simulink model "hiptourque"  (R2014b)
settings: Solver=ode3  StartTime=0.0  StopTime=4  FixedStep=.01  RelTol=1e-3
values from neighbouring files (symbols this model uses):
  k = 10    [hip.m]
  p = -phi(end)    [hip.m]
  p1 = (1-cos(phi(end)))*cos(phi(end))*thetadot(end)    [hip.m]
  t1 = cos(phi(end))*thetadot(end)    [hip.m]
settings Model: Creator=hamidreza  LastModifiedBy=hamidreza

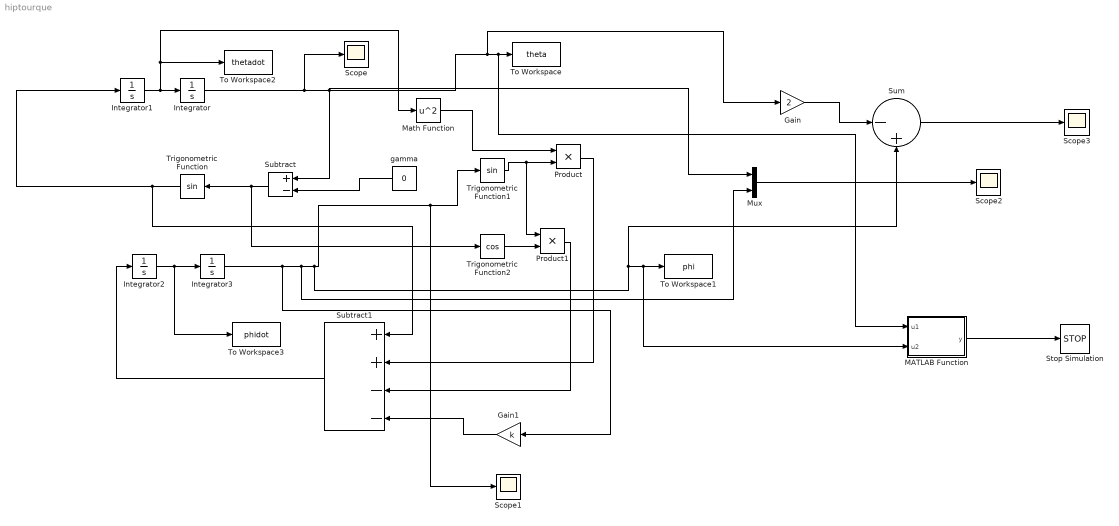
== system hiptourque ==
  Gain : Gain  Gain=2
  Gain1 : Gain  Gain=k
  Integrator : Integrator  InitialCondition=t
  Integrator1 : Integrator  InitialCondition=t1
  Integrator2 : Integrator  InitialCondition=p1
  Integrator3 : Integrator  InitialCondition=p
  MATLAB Function : MATLAB Function  TreatAsAtomicUnit=on
  Math Function : Math  Operator=square  SaturateOnIntegerOverflow=on
  Mux : Mux  Inputs=2
  Product : Product
  Product1 : Product
  Scope{,1..3} (4 alike) : Scope
      Scope1 settings: TimeRange=10  YMin=-1  YMax=1.5
      Scope2 settings: TimeRange=0.66  YMin=-0.2  YMax=0.2  SaveName=ScopeData2
      Scope3 settings: SaveName=ScopeData3
  Stop Simulation : Stop
  Subtract : Sum  Inputs=+-
  Subtract1 : Sum  Inputs=++--
  Sum : Sum  Inputs=|-+
  To Workspace : ToWorkspace  VariableName=theta  SaveFormat=Structure With Time  SampleTime=-1
  To Workspace1 : ToWorkspace  VariableName=phi  SaveFormat=Structure With Time  SampleTime=-1
  To Workspace2 : ToWorkspace  VariableName=thetadot  SaveFormat=Structure With Time  SampleTime=-1
  To Workspace3 : ToWorkspace  VariableName=phidot  SaveFormat=Structure With Time  SampleTime=-1
  Trigonometric Function : Trigonometry  OutputSignalType=real
  Trigonometric Function1 : Trigonometry
  Trigonometric Function2 : Trigonometry  Operator=cos
  "gamma " : Constant  Value=0
  wires:
  Integrator/1 -> Scope/1, Subtract/1, Mux/1, Gain/1, MATLAB Function/1(u1), To Workspace/1
  Trigonometric Function/1 -> Subtract1/1, Integrator1/1
  Integrator1/1 -> Math Function/1, To Workspace2/1, Integrator/1
  Integrator2/1 -> To Workspace3/1, Integrator3/1
  "gamma "/1 -> Subtract/2
  Subtract/1 -> Trigonometric Function2/1, Trigonometric Function/1
  Math Function/1 -> Product/1
  Integrator3/1 -> Gain1/1, Mux/2, Sum/2, MATLAB Function/2(u2), To Workspace1/1, Scope1/1, Trigonometric Function1/1
  Trigonometric Function1/1 -> Product1/1, Product/2
  Product/1 -> Subtract1/2
  Subtract1/1 -> Integrator2/1
  Trigonometric Function2/1 -> Product1/2
  Product1/1 -> Subtract1/3
  Mux/1 -> Scope2/1
  Gain/1 -> Sum/1
  Sum/1 -> Scope3/1
  MATLAB Function/1(y) -> Stop Simulation/1
  Gain1/1 -> Subtract1/4

== matlab function hiptourque/MATLAB Function ==
  data: u1 input; y output; u2 input
function y = fcn(u1,u2)
%#codegen

if and(u2<-.15,abs(u2-2*u1)<.007)
    y=1;
else
    y=0;
   
end
